simulink model "Enable_Subsystem_Constant_and_Pulse_Generator"  (R2024b)
settings: Solver=FixedStepAuto  StartTime=0.0  StopTime=10  FixedStep=0.1  RelTol=1e-3
settings Model: Creator=abdal  LastModifiedBy=abdal

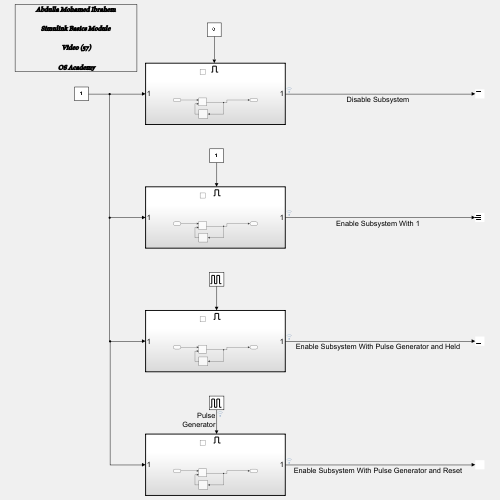
[thumbnail: Simulink's stored preview of the top-level diagram]
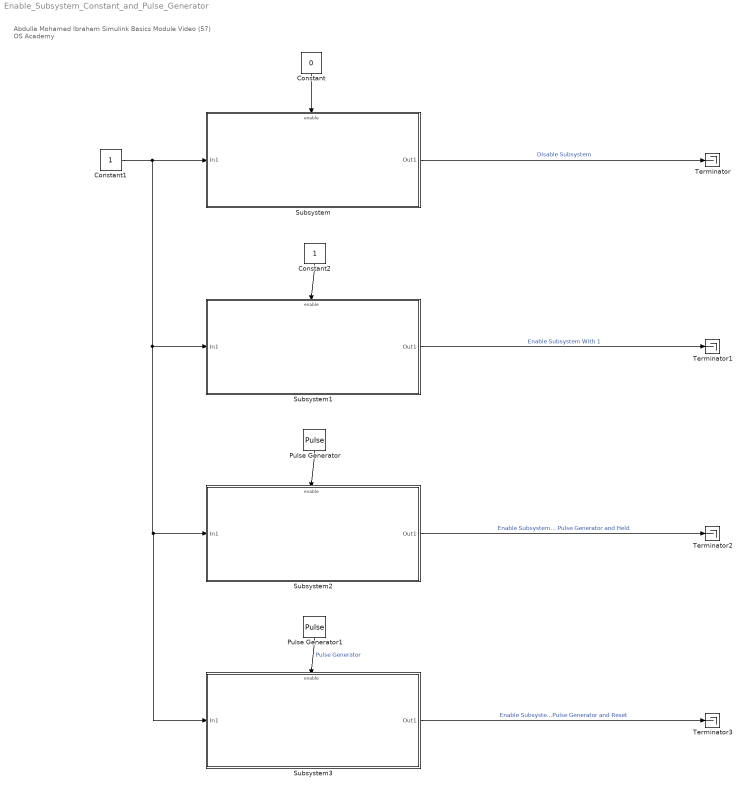
== system Enable_Subsystem_Constant_and_Pulse_Generator ==
  note: Abdulla Mohamed Ibrahem
      | Simulink Basics Module
      | Video (57)
      | OS Academy
  Constant : Constant  Value=0
  Constant1 : Constant
  Constant2 : Constant
  Pulse Generator : DiscretePulseGenerator  PulseType=Time based  PulseWidth=50
  Pulse Generator1 : DiscretePulseGenerator  PulseType=Time based  PulseWidth=50
  Subsystem : Subsystem  TreatAsAtomicUnit=on
  Subsystem1 : Subsystem  TreatAsAtomicUnit=on
  Subsystem2 : Subsystem  TreatAsAtomicUnit=on
  Subsystem3 : Subsystem  TreatAsAtomicUnit=on
  Terminator{,1..3} (4 alike) : Terminator
  wires:
  Constant/1 -> Subsystem/Enable
  Subsystem/1(Out1) -> Terminator/1  "Disable Subsystem"
  Constant2/1 -> Subsystem1/Enable
  Pulse Generator/1 -> Subsystem2/Enable
  Pulse Generator1/1 -> Subsystem3/Enable  "Pulse Generator"
  Constant1/1 -> Subsystem/1(In1), Subsystem3/1(In1), Subsystem2/1(In1), Subsystem1/1(In1)
  Subsystem1/1(Out1) -> Terminator1/1  "Enable Subsystem With 1"
  Subsystem2/1(Out1) -> Terminator2/1  "Enable Subsystem With Pulse Generator and Held"
  Subsystem3/1(Out1) -> Terminator3/1  "Enable Subsystem With Pulse Generator and Reset"

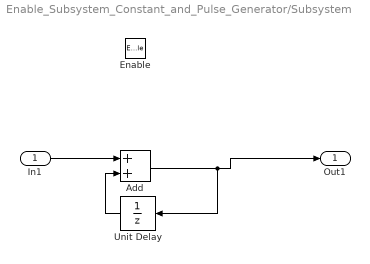
== system Enable_Subsystem_Constant_and_Pulse_Generator/Subsystem ==
  In1 : Inport
  Enable : EnablePort
  Add : Sum
  Unit Delay : UnitDelay  SampleTime=-1  HasFrameUpgradeWarning=on
  Out1 : Outport
  wires:
  In1/1 -> Add/1
  Add/1 -> Unit Delay/1, Out1/1
  Unit Delay/1 -> Add/2

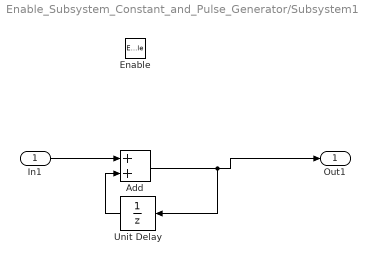
== system Enable_Subsystem_Constant_and_Pulse_Generator/Subsystem1 ==
  In1 : Inport
  Enable : EnablePort
  Add : Sum
  Unit Delay : UnitDelay  SampleTime=-1  HasFrameUpgradeWarning=on
  Out1 : Outport
  wires:
  Unit Delay/1 -> Add/2
  Add/1 -> Out1/1, Unit Delay/1
  In1/1 -> Add/1

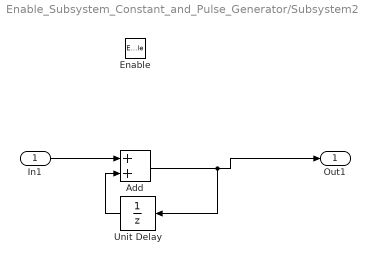
== system Enable_Subsystem_Constant_and_Pulse_Generator/Subsystem2 ==
  In1 : Inport
  Enable : EnablePort
  Add : Sum
  Unit Delay : UnitDelay  SampleTime=-1  HasFrameUpgradeWarning=on
  Out1 : Outport
  wires:
  In1/1 -> Add/1
  Add/1 -> Unit Delay/1, Out1/1
  Unit Delay/1 -> Add/2

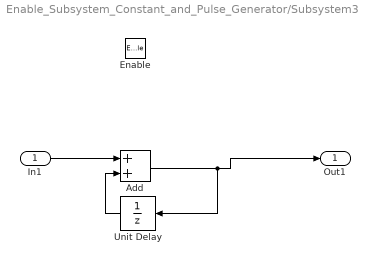
== system Enable_Subsystem_Constant_and_Pulse_Generator/Subsystem3 ==
  In1 : Inport
  Enable : EnablePort  StatesWhenEnabling=reset
  Add : Sum
  Unit Delay : UnitDelay  SampleTime=-1  HasFrameUpgradeWarning=on
  Out1 : Outport
  wires:
  Unit Delay/1 -> Add/2
  Add/1 -> Out1/1, Unit Delay/1
  In1/1 -> Add/1
